simulink model "gm_uz_pmsm_model_6LUT_pd"  (R2023b)
settings: Solver=FixedStepAuto  StartTime=0.0  StopTime=0.05  RelTol=1e-3
PreLoadFcn:
  | uz_pmsm_model_init_parameter
PostLoadFcn:
  | % Import the data from Excel for a lookup table
  | FluxMapData = readtable('C:\Users\Philipp\ultrazohm\ultrazohm_sw\ip_cores\uz_pmsm_model\FluxMapData_2023-05-26_13-07-57.csv');
  | % Row indices for lookup table
  | d_current_in_d_axis = FluxMapData(8:27,1:end);
  | % Column indices for lookup table
  | q_current_in_d_axis = FluxMapData(29:48,1:end);
  | % Output values for lookup table
  | d_Flux_d_axis = FluxMapData(50:69,1:end);
undefined symbols (not defined in the file or in its folder): ad1, ad2, ad3, ad4, ad5, ad6, aq1, aq2, aq3, aq4, aq5, aq6, d_current_d_Flux, d_current_q_Flux, entkopplung_dynamic, entkopplung_linear, entkopplung_static, Fid1_Giq1, Fid2_Giq2, Flux_d, Flux_q, friction_coefficient, inertia, Ki_Bo_d, Ki_Bo_q, Kp_Bo_d, Kp_Bo_q, L_d, L_q, Ldq, parameter_nachfuerung, polepair, praediktion_entkopplung_nonlinear, psi_pm, q_current_d_Flux, q_current_q_Flux, R_1, simulate_mechanical, simulate_nonlinear_modell, simulate_open_loop, static_friction_torque, tau_sum, ts_regler
libraries: hdlmdlgenlib x21, slpidlib x2
(part 2 of 3)

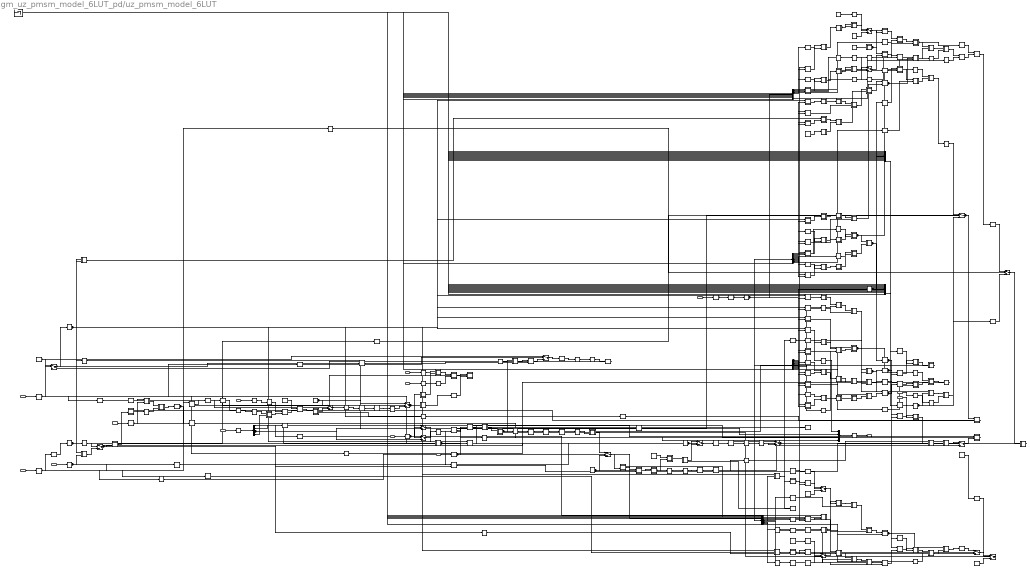
== system gm_uz_pmsm_model_6LUT_pd/uz_pmsm_model_6LUT ==
  reset_integrators : Inport  OutDataTypeStr=boolean  PortDimensions=1  SampleTime=2e-06
  simulate_mechanical : Inport  Port=2  OutDataTypeStr=boolean  PortDimensions=1  SampleTime=2e-06
  simulate_nonlinear : Inport  Port=3  OutDataTypeStr=boolean  PortDimensions=1  SampleTime=2e-06
  reciprocal_J : Inport  Port=4  OutDataTypeStr=single  PortDimensions=1  SampleTime=2e-06
  mu : Inport  Port=5  OutDataTypeStr=single  PortDimensions=1  SampleTime=2e-06
  M_n0 : Inport  Port=6  OutDataTypeStr=single  PortDimensions=1  SampleTime=2e-06
  R1 : Inport  Port=7  OutDataTypeStr=single  PortDimensions=1  SampleTime=2e-06
  polepairs : Inport  Port=8  OutDataTypeStr=single  PortDimensions=1  SampleTime=2e-06
  Ld : Inport  Port=9  OutDataTypeStr=single  PortDimensions=1  SampleTime=2e-06
  Lq : Inport  Port=10  OutDataTypeStr=single  PortDimensions=1  SampleTime=2e-06
  psi_pm : Inport  Port=11  OutDataTypeStr=single  PortDimensions=1  SampleTime=2e-06
  fitting_parameters : Inport  Port=12  OutDataTypeStr=single  PortDimensions=[14]  SampleTime=2e-06
  inputs : Inport  Port=13  OutDataTypeStr=single  PortDimensions=[4]  SampleTime=2e-06
  Abs : Subsystem
      mask Display: disp('NFP\nabs');
  Constant : Constant  Value=double(0.5)  OutDataTypeStr=double  SampleTime=1e-08
  Constant1 : Constant  Value=double(1)  OutDataTypeStr=double  SampleTime=1e-08
  Constant11 : Constant  Value=double(1)  OutDataTypeStr=double  SampleTime=1e-08
  Data Type Conversion{11,15..17} (4 alike) : DataTypeConversion  OutDataTypeStr=single
  Data Type Conversion171 : Subsystem
      mask Display: disp('NFP\nconv');
  Data Type Conversion172 : Subsystem
      mask Display: disp('NFP\nconv');
  Data Type Conversion173 : Subsystem
      mask Display: disp('NFP\nconv');
  Data Type Conversion17_to_const : Constant  Value=double(0)  OutDataTypeStr=single  SampleTime=1e-08
  Delay : RateTransition  OutPortSampleTimeOpt=Multiple of input port sample time  OutPortSampleTimeMultiple=200
  Delay1_lowered : RateTransition  OutPortSampleTimeOpt=Multiple of input port sample time  OutPortSampleTimeMultiple=200
  Delay1_lowered1 : RateTransition  OutPortSampleTimeOpt=Multiple of input port sample time  OutPortSampleTimeMultiple=200
  Delay1_lowered2 : RateTransition  OutPortSampleTimeOpt=Multiple of input port sample time  OutPortSampleTimeMultiple=200
  Delay1_lowered_absorbed : Delay  DelayLength=0
  Delay1_lowered_absorbed1 : Delay  DelayLength=0
  Delay1_lowered_absorbed2 : Delay  DelayLength=0
  Delay_absorbed : Delay  DelayLength=0
  Divide : Subsystem
      mask Display: disp('NFP\nmul');
  Divide1 : Subsystem
      mask Display: disp('NFP\nmul');
  Divide_recip : Subsystem
      mask Display: disp('NFP\nmath');
  Factor : Subsystem
      mask Display: disp('NFP\nmul');
  Factor_const : Constant  Value=single(1.5)  OutDataTypeStr=single  SampleTime=1e-08
  From1 : hdlmdlgenlib/Buffer
  From1_out1_0_term0 : Terminator
  From1_out1_10_term10 : Terminator
  From1_out1_11_term11 : Terminator
  From1_out1_12_term12 : Terminator
  From1_out1_13_term13 : Terminator
  From1_out1_1_term1 : Terminator
  From1_out1_2_term2 : Terminator
  From1_out1_3_term3 : Terminator
  From1_out1_4_term4 : Terminator
  From1_out1_5_term5 : Terminator
  From1_out1_6_term6 : Terminator
  From1_out1_7_term7 : Terminator
  From1_out1_8_term8 : Terminator
  From1_out1_9_term9 : Terminator
  From2 : hdlmdlgenlib/Buffer
  From2_out1_0_term0 : Terminator
  From2_out1_0_term01 : Terminator
  From2_out1_10_term10 : Terminator
  From2_out1_10_term101 : Terminator
  From2_out1_11_term11 : Terminator
  From2_out1_11_term111 : Terminator
  From2_out1_12_term12 : Terminator
  From2_out1_13_term13 : Terminator
  From2_out1_1_term1 : Terminator
  From2_out1_1_term11 : Terminator
  From2_out1_2_term2 : Terminator
  From2_out1_2_term21 : Terminator
  From2_out1_3_term3 : Terminator
  From2_out1_3_term31 : Terminator
  From2_out1_4_term4 : Terminator
  From2_out1_4_term41 : Terminator
  From2_out1_5_term5 : Terminator
  From2_out1_5_term51 : Terminator
  From2_out1_6_term6 : Terminator
  From2_out1_6_term61 : Terminator
  From2_out1_7_term7 : Terminator
  From2_out1_7_term71 : Terminator
  From2_out1_8_term8 : Terminator
  From2_out1_8_term81 : Terminator
  From2_out1_9_term9 : Terminator
  From2_out1_9_term91 : Terminator
  From3 : hdlmdlgenlib/Buffer
  Gain : Subsystem
      mask Display: disp('NFP\nmul');
  Gain7 : Subsystem
      mask Display: disp('NFP\nmul');
  Gain71 : Subsystem
      mask Display: disp('NFP\nmul');
  Gain7_const : Constant  Value=single(2e-06)  OutDataTypeStr=single  SampleTime=1e-08
  Gain7_const1 : Constant  Value=single(2e-06)  OutDataTypeStr=single  SampleTime=1e-08
  Gain_const : Constant  Value=single(2e-06)  OutDataTypeStr=single  SampleTime=1e-08
  Gain_unaryminus : Subsystem
      mask Display: disp('NFP\numinus');
  Gain_unaryminus1 : Subsystem
      mask Display: disp('NFP\numinus');
  Goto1 : hdlmdlgenlib/Buffer
  Goto2 : hdlmdlgenlib/Buffer
  Initial_Val : Constant  Value=single(0)  OutDataTypeStr=single  SampleTime=1e-08
  Initial_Val1 : Constant  Value=single(0)  OutDataTypeStr=single  SampleTime=1e-08
  Initial_Val2 : Constant  Value=single(0)  OutDataTypeStr=single  SampleTime=1e-08
  Ldd : hdlmdlgenlib/Buffer
  Log : Subsystem
      mask Display: disp('NFP\nmath');
  Log1 : Subsystem
      mask Display: disp('NFP\nmath');
  Log11 : Subsystem
      mask Display: disp('NFP\nmath');
  Log2 : Subsystem
      mask Display: disp('NFP\nmath');
  Lqq : hdlmdlgenlib/Buffer
  M_Mi : hdlmdlgenlib/Buffer
  Product : Subsystem
      mask Display: disp('NFP\nmul');
  Product1 : Subsystem
      mask Display: disp('NFP\nmul');
  Product10 : Subsystem
      mask Display: disp('NFP\nmul');
  Product101 : Subsystem
      mask Display: disp('NFP\nmul');
  Product102 : Subsystem
      mask Display: disp('NFP\nmul');
  Product103 : Subsystem
      mask Display: disp('NFP\nmul');
  Product104 : Subsystem
      mask Display: disp('NFP\nmul');
  Product11 : Subsystem
      mask Display: disp('NFP\nmul');
  Product110 : Subsystem
      mask Display: disp('NFP\nmul');
  Product111 : Subsystem
      mask Display: disp('NFP\nmul');
  Product112 : Subsystem
      mask Display: disp('NFP\nmul');
  Product113 : Subsystem
      mask Display: disp('NFP\nmul');
  Product12 : Subsystem
      mask Display: disp('NFP\nmul');
  Product121 : Subsystem
      mask Display: disp('NFP\nmul');
  Product122 : Subsystem
      mask Display: disp('NFP\nmul');
  Product13 : Subsystem
      mask Display: disp('NFP\nmul');
  Product131 : Subsystem
      mask Display: disp('NFP\nmul');
  Product132 : Subsystem
      mask Display: disp('NFP\nmul');
  Product133 : Subsystem
      mask Display: disp('NFP\nmul');
  Product14 : Subsystem
      mask Display: disp('NFP\nmul');
  Product141 : Subsystem
      mask Display: disp('NFP\nmul');
  Product15 : Subsystem
      mask Display: disp('NFP\nmul');
  Product151 : Subsystem
      mask Display: disp('NFP\nmul');
  Product16 : Subsystem
      mask Display: disp('NFP\nmul');
  Product161 : Subsystem
      mask Display: disp('NFP\nmul');
  Product162 : Subsystem
      mask Display: disp('NFP\nmul');
  Product17 : Subsystem
      mask Display: disp('NFP\nmul');
  Product18 : Subsystem
      mask Display: disp('NFP\nmul');
  Product19 : Subsystem
      mask Display: disp('NFP\nmul');
  Product2 : Subsystem
      mask Display: disp('NFP\nmul');
  Product20 : Subsystem
      mask Display: disp('NFP\nmul');
  Product201 : Subsystem
      mask Display: disp('NFP\nmul');
  Product202 : Subsystem
      mask Display: disp('NFP\nmul');
  Product203 : Subsystem
      mask Display: disp('NFP\nmul');
  Product204 : Subsystem
      mask Display: disp('NFP\nmul');
  Product205 : Subsystem
      mask Display: disp('NFP\nmul');
  Product206 : Subsystem
      mask Display: disp('NFP\nmul');
  Product207 : Subsystem
      mask Display: disp('NFP\nmul');
  Product21 : Subsystem
      mask Display: disp('NFP\nmul');
  Product211 : Subsystem
      mask Display: disp('NFP\nmul');
  Product22 : Subsystem
      mask Display: disp('NFP\nmul');
  Product23 : Subsystem
      mask Display: disp('NFP\nmul');
  Product24 : Subsystem
      mask Display: disp('NFP\nmul');
  Product25 : Subsystem
      mask Display: disp('NFP\nmul');
  Product26 : Subsystem
      mask Display: disp('NFP\nmul');
  Product3 : Subsystem
      mask Display: disp('NFP\nmul');
  Product31 : Subsystem
      mask Display: disp('NFP\nmul');
  Product32 : Subsystem
      mask Display: disp('NFP\nmul');
  Product33 : Subsystem
      mask Display: disp('NFP\nmul');
  Product34 : Subsystem
      mask Display: disp('NFP\nmul');
  Product35 : Subsystem
      mask Display: disp('NFP\nmul');
  Product36 : Subsystem
      mask Display: disp('NFP\nmul');
  Product37 : Subsystem
      mask Display: disp('NFP\nmul');
  Product4 : Subsystem
      mask Display: disp('NFP\nmul');
  Product41 : Subsystem
      mask Display: disp('NFP\nmul');
  Product42 : Subsystem
      mask Display: disp('NFP\nmul');
  Product43 : Subsystem
      mask Display: disp('NFP\nmul');
  Product44 : Subsystem
      mask Display: disp('NFP\nmul');
  Product5 : Subsystem
      mask Display: disp('NFP\nmul');
  Product51 : Subsystem
      mask Display: disp('NFP\nmul');
  Product52 : Subsystem
      mask Display: disp('NFP\nmul');
  Product6 : Subsystem
      mask Display: disp('NFP\nmul');
  Product61 : Subsystem
      mask Display: disp('NFP\nmul');
  Product7 : Subsystem
      mask Display: disp('NFP\nmul');
  Product71 : Subsystem
      mask Display: disp('NFP\nmul');
  Product72 : Subsystem
      mask Display: disp('NFP\nmul');
  Product8 : Subsystem
      mask Display: disp('NFP\nmul');
  Product81 : Subsystem
      mask Display: disp('NFP\nmul');
  Product9 : Subsystem
      mask Display: disp('NFP\nmul');
  Product91 : Subsystem
      mask Display: disp('NFP\nmul');
  Product92 : Subsystem
      mask Display: disp('NFP\nmul');
  Product93 : Subsystem
      mask Display: disp('NFP\nmul');
  Sign1 : Subsystem
      mask Display: disp('NFP\nsignum');
  Sum : Subsystem
      mask Display: disp('NFP\nadd');
  Sum1 : Subsystem
      mask Display: disp('NFP\nadd');
  Sum10 : Subsystem
      mask Display: disp('NFP\nadd');
  Sum101 : Subsystem
      mask Display: disp('NFP\nadd');
  Sum11 : Subsystem
      mask Display: disp('NFP\nadd');
  Sum12 : Subsystem
      mask Display: disp('NFP\nadd');
  Sum13 : Subsystem
      mask Display: disp('NFP\nadd');
  Sum14 : Subsystem
      mask Display: disp('NFP\nadd');
  Sum2 : Subsystem
      mask Display: disp('NFP\nadd');
  Sum21 : Subsystem
      mask Display: disp('NFP\nadd');
  Sum22 : Subsystem
      mask Display: disp('NFP\nadd');
  Sum23 : Subsystem
      mask Display: disp('NFP\nadd');
  Sum3 : Subsystem
      mask Display: disp('NFP\nadd');
  Sum31 : Subsystem
      mask Display: disp('NFP\nadd');
  Sum32 : Subsystem
      mask Display: disp('NFP\nadd');
  Sum33 : Subsystem
      mask Display: disp('NFP\nadd');
  Sum3_stage2 : Subsystem
      mask Display: disp('NFP\nadd');
  Sum3_stage21 : Subsystem
      mask Display: disp('NFP\nadd');
  Sum3_stage3 : Subsystem
      mask Display: disp('NFP\nadd');
  Sum3_stage31 : Subsystem
      mask Display: disp('NFP\nadd');
  Sum3_stage4 : Subsystem
      mask Display: disp('NFP\nadd');
  Sum4 : Subsystem
      mask Display: disp('NFP\nadd');
  Sum41 : Subsystem
      mask Display: disp('NFP\nadd');
  Sum42 : Subsystem
      mask Display: disp('NFP\nadd');
  Sum43 : Subsystem
      mask Display: disp('NFP\nadd');
  Sum4_stage2 : Subsystem
      mask Display: disp('NFP\nadd');
  Sum4_stage3 : Subsystem
      mask Display: disp('NFP\nadd');
  Sum4_stage4 : Subsystem
      mask Display: disp('NFP\nadd');
  Sum5 : Subsystem
      mask Display: disp('NFP\nadd');
  Sum51 : Subsystem
      mask Display: disp('NFP\nadd');
  Sum52 : Subsystem
      mask Display: disp('NFP\nadd');
  Sum53 : Subsystem
      mask Display: disp('NFP\nadd');
  Sum6 : Subsystem
      mask Display: disp('NFP\nadd');
  Sum7 : Subsystem
      mask Display: disp('NFP\nadd');
  Sum71 : Subsystem
      mask Display: disp('NFP\nadd');
  Sum8 : Subsystem
      mask Display: disp('NFP\nadd');
  Switch{,1..6,11} (8 alike) : Switch  Criteria=u2 ~= 0  Threshold=double(0)  OutDataTypeStr=single  SampleTime=1e-08  SaturateOnIntegerOverflow=off  InputSameDT=off
  Tanh : Subsystem
      mask Display: disp('NFP\ntrig');
  Tanh1 : Subsystem
      mask Display: disp('NFP\ntrig');
  Tanh11 : Subsystem
      mask Display: disp('NFP\ntrig');
  Tanh12 : Subsystem
      mask Display: disp('NFP\ntrig');
  Tanh13 : Subsystem
      mask Display: disp('NFP\ntrig');
  Tanh2 : Subsystem
      mask Display: disp('NFP\ntrig');
  Tanh21 : Subsystem
      mask Display: disp('NFP\ntrig');
  Tanh3 : Subsystem
      mask Display: disp('NFP\ntrig');
  Tanh31 : Subsystem
      mask Display: disp('NFP\ntrig');
  Tanh4 : Subsystem
      mask Display: disp('NFP\ntrig');
  Tanh41 : Subsystem
      mask Display: disp('NFP\ntrig');
  Tanh5 : Subsystem
      mask Display: disp('NFP\ntrig');
  Unit Delay : RateTransition  OutPortSampleTimeOpt=Multiple of input port sample time  OutPortSampleTimeMultiple=200
  Unit Delay1 : RateTransition  OutPortSampleTimeOpt=Multiple of input port sample time  OutPortSampleTimeMultiple=200
  Unit Delay1_absorbed : Delay  DelayLength=0
  Unit Delay_absorbed : Delay  DelayLength=0
  crp_out_delay{,1..5} (6 alike) : Delay  DelayLength=double(1)  InitialCondition=0  SampleTime=1e-08
  default_value{,1..4} (5 alike) : Constant  Value=double(1)  OutDataTypeStr=single  SampleTime=1e-08
  delayMatch{,1..24,26..28,30..41,43..45,47..52,54..58} (54 alike) : Delay  DelayLength=double(1)  InitialCondition=0  SampleTime=1e-08
  delayMatch25 : Delay  DelayLength=double(35)  InitialCondition=0  SampleTime=1e-08
  delayMatch29 : Delay  DelayLength=double(35)  InitialCondition=0  SampleTime=1e-08
  delayMatch42 : Delay  DelayLength=double(29)  InitialCondition=0  SampleTime=1e-08
  delayMatch46 : Delay  DelayLength=double(29)  InitialCondition=0  SampleTime=1e-08
  delayMatch53 : Delay  DelayLength=double(97)  InitialCondition=0  SampleTime=1e-08
  fitting_parameters_12_term12 : Terminator
  fitting_parameters_13_term13 : Terminator
  in0_repeat : RateTransition  Integrity=off  Deterministic=off  OutPortSampleTimeOpt=Multiple of input port sample time  OutPortSampleTimeMultiple=1/200
  in10_repeat : RateTransition  Integrity=off  Deterministic=off  OutPortSampleTimeOpt=Multiple of input port sample time  OutPortSampleTimeMultiple=1/200
  in11_repeat : RateTransition  Integrity=off  Deterministic=off  OutPortSampleTimeOpt=Multiple of input port sample time  OutPortSampleTimeMultiple=1/200
  in12_repeat : RateTransition  Integrity=off  Deterministic=off  OutPortSampleTimeOpt=Multiple of input port sample time  OutPortSampleTimeMultiple=1/200
  in13_repeat : RateTransition  Integrity=off  Deterministic=off  OutPortSampleTimeOpt=Multiple of input port sample time  OutPortSampleTimeMultiple=1/200
  in14_repeat : RateTransition  Integrity=off  Deterministic=off  OutPortSampleTimeOpt=Multiple of input port sample time  OutPortSampleTimeMultiple=1/200
  in15_repeat : RateTransition  Integrity=off  Deterministic=off  OutPortSampleTimeOpt=Multiple of input port sample time  OutPortSampleTimeMultiple=1/200
  in16_repeat : RateTransition  Integrity=off  Deterministic=off  OutPortSampleTimeOpt=Multiple of input port sample time  OutPortSampleTimeMultiple=1/200
  in17_repeat : RateTransition  Integrity=off  Deterministic=off  OutPortSampleTimeOpt=Multiple of input port sample time  OutPortSampleTimeMultiple=1/200
  in18_repeat : RateTransition  Integrity=off  Deterministic=off  OutPortSampleTimeOpt=Multiple of input port sample time  OutPortSampleTimeMultiple=1/200
  in1_repeat : RateTransition  Integrity=off  Deterministic=off  OutPortSampleTimeOpt=Multiple of input port sample time  OutPortSampleTimeMultiple=1/200
  in2_repeat : RateTransition  Integrity=off  Deterministic=off  OutPortSampleTimeOpt=Multiple of input port sample time  OutPortSampleTimeMultiple=1/200
  in3_repeat : RateTransition  Integrity=off  Deterministic=off  OutPortSampleTimeOpt=Multiple of input port sample time  OutPortSampleTimeMultiple=1/200
  in4_repeat : RateTransition  Integrity=off  Deterministic=off  OutPortSampleTimeOpt=Multiple of input port sample time  OutPortSampleTimeMultiple=1/200
  in5_repeat : RateTransition  Integrity=off  Deterministic=off  OutPortSampleTimeOpt=Multiple of input port sample time  OutPortSampleTimeMultiple=1/200
  in6_repeat : RateTransition  Integrity=off  Deterministic=off  OutPortSampleTimeOpt=Multiple of input port sample time  OutPortSampleTimeMultiple=1/200
  in7_repeat : RateTransition  Integrity=off  Deterministic=off  OutPortSampleTimeOpt=Multiple of input port sample time  OutPortSampleTimeMultiple=1/200
  in8_repeat : RateTransition  Integrity=off  Deterministic=off  OutPortSampleTimeOpt=Multiple of input port sample time  OutPortSampleTimeMultiple=1/200
  in9_repeat : RateTransition  Integrity=off  Deterministic=off  OutPortSampleTimeOpt=Multiple of input port sample time  OutPortSampleTimeMultiple=1/200
  mux : Mux
  psi_d_approx : hdlmdlgenlib/Buffer
  psi_q_approx : hdlmdlgenlib/Buffer
  reset_in : Switch  Criteria=u2 ~= 0  Threshold=double(0)  OutDataTypeStr=single  SampleTime=1e-08  SaturateOnIntegerOverflow=off  InputSameDT=off
  reset_in1 : Switch  Criteria=u2 ~= 0  Threshold=double(0)  OutDataTypeStr=single  SampleTime=1e-08  SaturateOnIntegerOverflow=off  InputSameDT=off
  reset_in2 : Switch  Criteria=u2 ~= 0  Threshold=double(0)  OutDataTypeStr=single  SampleTime=1e-08  SaturateOnIntegerOverflow=off  InputSameDT=off
  reset_out : Switch  Criteria=u2 ~= 0  Threshold=double(0)  OutDataTypeStr=single  SampleTime=1e-08  SaturateOnIntegerOverflow=off  InputSameDT=off
  reset_out1 : Switch  Criteria=u2 ~= 0  Threshold=double(0)  OutDataTypeStr=single  SampleTime=1e-08  SaturateOnIntegerOverflow=off  InputSameDT=off
  reset_out2 : Switch  Criteria=u2 ~= 0  Threshold=double(0)  OutDataTypeStr=single  SampleTime=1e-08  SaturateOnIntegerOverflow=off  InputSameDT=off
  select_signal{,1..4} (5 alike) : Constant  Value=double(1)  OutDataTypeStr=boolean  SampleTime=1e-08
  t : RateTransition  OutPortSampleTimeOpt=Multiple of input port sample time  OutPortSampleTimeMultiple=200
  t{1..6} (6 alike) : Demux  Outputs=14
  t{8..18} (11 alike) : hdlmdlgenlib/Buffer
  t7 : Demux
  zero_protection{,1..4} (5 alike) : Switch  Criteria=u2 ~= 0  Threshold=double(0)  OutDataTypeStr=single  SampleTime=1e-08  SaturateOnIntegerOverflow=off  InputSameDT=off
  outputs : Outport  SampleTime=2e-06
  wires:
  reset_integrators/1 -> in8_repeat/1
  simulate_mechanical/1 -> in10_repeat/1
  simulate_nonlinear/1 -> in1_repeat/1
  reciprocal_J/1 -> in12_repeat/1
  mu/1 -> in0_repeat/1
  M_n0/1 -> in18_repeat/1
  R1/1 -> in3_repeat/1
  polepairs/1 -> in17_repeat/1
  Ld/1 -> in4_repeat/1
  Lq/1 -> in2_repeat/1
  psi_pm/1 -> in5_repeat/1
  fitting_parameters/1 -> in7_repeat/1
  inputs/1 -> in14_repeat/1
  t/1 -> outputs/1
  in0_repeat/1 -> Product122/1(In1)
  in1_repeat/1 -> delayMatch51/1, delayMatch40/1, delayMatch34/1, delayMatch33/1, Goto2/1
  in2_repeat/1 -> delayMatch52/1, Product1/2(In2)
  in3_repeat/1 -> Product43/1(In1), Product9/2(In2)
  in4_repeat/1 -> delayMatch35/1, Product5/2(In2)
  in5_repeat/1 -> delayMatch5/1
  in7_repeat/1 -> t6/1, t3/1, Goto1/1
  in8_repeat/1 -> delayMatch58/1, delayMatch55/1, delayMatch37/1, reset_out1/2, reset_out2/2, reset_out/2
  in10_repeat/1 -> Switch/2, Switch11/2
  in12_repeat/1 -> delayMatch56/1
  in14_repeat/1 -> t7/1
  in17_repeat/1 -> delayMatch15/1, Product131/2(In2)
  in18_repeat/1 -> delayMatch19/1
  mux/1 -> t/1
  Delay1_lowered/1 -> Delay1_lowered_absorbed/1
  Delay1_lowered_absorbed/1 -> in16_repeat/1
  in16_repeat/1 -> reset_out2/3
  Unit Delay1/1 -> Unit Delay1_absorbed/1
  Unit Delay1_absorbed/1 -> in15_repeat/1
  in15_repeat/1 -> delayMatch23/1
  Delay/1 -> Delay_absorbed/1
  Delay_absorbed/1 -> in13_repeat/1
  in13_repeat/1 -> Sum14/1(In1)
  Delay1_lowered1/1 -> Delay1_lowered_absorbed1/1
  Delay1_lowered_absorbed1/1 -> in11_repeat/1
  in11_repeat/1 -> reset_out1/3
  Delay1_lowered2/1 -> Delay1_lowered_absorbed2/1
  Delay1_lowered_absorbed2/1 -> in9_repeat/1
  in9_repeat/1 -> reset_out/3
  Unit Delay/1 -> Unit Delay_absorbed/1
  Unit Delay_absorbed/1 -> in6_repeat/1
  in6_repeat/1 -> delayMatch39/1
  crp_out_delay/1 -> Delay/1
  crp_out_delay1/1 -> Unit Delay/1
  crp_out_delay2/1 -> Delay1_lowered/1
  crp_out_delay3/1 -> Unit Delay1/1
  crp_out_delay4/1 -> Delay1_lowered2/1
  crp_out_delay5/1 -> Delay1_lowered1/1
  Data Type Conversion16/1 -> mux/3
  Lqq/1 -> Switch1/1
  Constant1/1 -> Data Type Conversion171/1(In1)
  Data Type Conversion171/1(Out1) -> Product133/1(In1), Product162/1(In1)
  Switch2/1 -> Divide_recip/1(In1)
  Ldd/1 -> Switch2/1
  Constant11/1 -> Data Type Conversion172/1(In1)
  Data Type Conversion172/1(Out1) -> Product132/1(In1), Product161/1(In1)
  Product31/1(Out1) -> Sum2/2(In2)
  Sum2/1(Out1) -> Product102/1(In1)
  Product21/1(Out1) -> Sum4_stage3/2(In2)
  Goto2/1 -> From3/1
  delayMatch6/1 -> Switch5/2
  Switch5/1 -> Product21/1(In1), Product37/1(In1)
  psi_d_approx/1 -> Switch5/1
  Gain_unaryminus/1(Out1) -> Product11/2(In2)
  delayMatch22/1 -> Product207/2(In2)
  Goto1/1 -> From2/1, From1/1
  From2/1 -> t2/1, t1/1
  delayMatch38/1 -> Product201/2(In2)
  Product201/1(Out1) -> Gain_unaryminus/1(In1)
  t10/1 -> Product206/1(In1), Product20/1(In1)
  Constant/1 -> Data Type Conversion173/1(In1)
  Data Type Conversion173/1(Out1) -> Product71/2(In2)
  Sum41/1(Out1) -> Product7/2(In2)
  delayMatch1/1 -> Product13/2(In2)
  delayMatch/1 -> Product4/2(In2)
  t3/3 -> Sum4/2(In2)
  delayMatch3/1 -> Product32/2(In2)
  delayMatch2/1 -> Product22/2(In2)
  t3/6 -> Sum11/2(In2)
  t3/7 -> Product93/1(In1)
  t3/8 -> Product41/2(In2), Product93/2(In2)
  t3/9 -> Sum41/1(In1)
  t3/10 -> Product113/1(In1)
  t3/11 -> Product51/2(In2), Product113/2(In2)
  t3/12 -> Sum41/2(In2)
  delayMatch4/1 -> Product101/2(In2)
  Product32/1(Out1) -> Sum21/2(In2)
  t15/1 -> Product10/1(In1)
  t14/1 -> Sum7/1(In1)
  Sum7/1(Out1) -> psi_d_approx/1
  Product101/1(Out1) -> Sum7/2(In2)
  Sum3_stage3/1(Out1) -> t8/1, Product10/2(In2)
  t8/1 -> Product102/2(In2)
  Product103/1(Out1) -> Sum71/2(In2)
  Sum71/1(Out1) -> Ldd/1
  t18/1 -> Sum71/1(In1)
  delayMatch26/1 -> Product16/2(In2)
  delayMatch24/1 -> Product/2(In2)
  t4/3 -> Sum/2(In2)
  delayMatch30/1 -> Product3/2(In2)
  delayMatch28/1 -> Product2/2(In2)
  t4/6 -> Sum1/2(In2)
  delayMatch32/1 -> Product103/2(In2)
  From1/1 -> t5/1, t4/1
  delayMatch43/1 -> Product19/2(In2)
  delayMatch44/1 -> Product110/2(In2)
  delayMatch45/1 -> Sum12/2(In2)
  delayMatch47/1 -> Product34/2(In2)
  delayMatch48/1 -> Product35/2(In2)
  delayMatch49/1 -> Sum42/2(In2)
  delayMatch50/1 -> Product205/2(In2)
  Product110/1(Out1) -> Sum12/1(In1)
  Sum10/1(Out1) -> Lqq/1
  Sum31/1(Out1) -> Product72/2(In2)
  Product72/1(Out1) -> Tanh41/1(In1)
  Sum6/1(Out1) -> Product104/2(In2)
  Product104/1(Out1) -> Tanh21/1(In1)
  Product33/1(Out1) -> Sum13/1(In1)
  t6/1 -> Product211/1(In1)
  delayMatch9/1 -> Product72/1(In1)
  t6/3 -> Sum31/2(In2)
  t6/4 -> Product81/1(In1)
  delayMatch10/1 -> Product104/1(In1)
  t6/6 -> Sum6/2(In2)
  delayMatch7/1 -> Product111/2(In2)
  t6/8 -> Product23/2(In2)
  t6/9 -> Product52/2(In2)
  delayMatch8/1 -> Product33/2(In2)
  t6/11 -> Product24/2(In2)
  t6/12 -> Product61/2(In2)
  delayMatch11/1 -> Product203/2(In2)
  Product203/1(Out1) -> Sum101/2(In2)
  Sum5/1(Out1) -> t9/1, Product202/2(In2)
  t9/1 -> Product204/2(In2)
  Product205/1(Out1) -> Sum10/2(In2)
  Product35/1(Out1) -> Sum42/1(In1)
  t11/1 -> Product25/1(In1), Product24/1(In1), Product61/1(In1), Product52/1(In1), Product23/1(In1), Product18/1(In1), Product51/1(In1), Product8/2(In2), Product8/1(In1), Product41/1(In1), Product9/1(In1), Product1/1(In1), delayMatch13/1, Data Type Conversion15/1
  delayMatch54/1 -> Sum51/2(In2)
  Initial_Val/1 -> reset_out/1, reset_in/1
  reset_in/1 -> crp_out_delay4/1
  Gain7/1(Out1) -> Sum51/1(In1)
  Divide1/1(Out1) -> Gain7/2(In2), crp_out_delay3/1
  delayMatch18/1 -> mux/4
  Switch11/1 -> Data Type Conversion17/1
  delayMatch57/1 -> Sum32/2(In2)
  Initial_Val1/1 -> reset_out1/1, reset_in1/1
  reset_in1/1 -> crp_out_delay5/1
  delayMatch21/1 -> Sum3_stage21/1(In1)
  delayMatch41/1 -> Sum4_stage2/1(In1)
  t7/3 -> Switch/3, Switch11/3
  t7/4 -> Sum14/2(In2)
  Switch4/1 -> Sum4_stage2/2(In2)
  Data Type Conversion17_to_const/1 -> Switch3/3, Switch4/3
  Switch3/1 -> Sum3_stage31/2(In2)
  Gain_unaryminus1/1(Out1) -> Product121/1(In1)
  Product207/1(Out1) -> Gain_unaryminus1/1(In1)
  t12/1 -> Product206/2(In2), Product20/2(In2)
  t16/1 -> Product202/1(In1)
  t17/1 -> Sum101/1(In1)
  Sum101/1(Out1) -> psi_q_approx/1
  psi_q_approx/1 -> Switch6/1
  Switch6/1 -> Product36/2(In2), Product26/2(In2)
  delayMatch14/1 -> Product26/1(In1)
  t13/1 -> Product43/2(In2), Sum6/1(In1), Sum31/1(In1), Sum11/1(In1), Sum4/1(In1), Product5/1(In1), Sum1/1(In1), Sum/1(In1), delayMatch14/1, Data Type Conversion11/1
  delayMatch36/1 -> Sum52/2(In2)
  Initial_Val2/1 -> reset_out2/1, reset_in2/1
  reset_in2/1 -> crp_out_delay2/1
  Gain71/1(Out1) -> Sum52/1(In1)
  Divide/1(Out1) -> Gain71/2(In2), crp_out_delay1/1
  Product36/1(Out1) -> Sum3_stage4/2(In2)
  Switch/1 -> Product131/1(In1)
  delayMatch20/1 -> Product44/2(In2)
  M_Mi/1 -> Sum8/1(In1), Data Type Conversion16/1
  Product92/1(Out1) -> M_Mi/1
  Factor/1(Out1) -> Product92/1(In1)
  delayMatch13/1 -> Product37/2(In2)
  delayMatch17/1 -> mux/2
  delayMatch16/1 -> mux/1
  delayMatch33/1 -> Switch3/2
  delayMatch52/1 -> Switch1/3
  delayMatch35/1 -> Switch2/3
  delayMatch5/1 -> Sum3/2(In2)
  delayMatch39/1 -> Product11/1(In1)
  delayMatch37/1 -> reset_in2/2
  delayMatch56/1 -> Product112/1(In1)
  delayMatch23/1 -> Product121/2(In2)
  delayMatch15/1 -> Product92/2(In2)
  delayMatch19/1 -> Sum53/2(In2)
  t1/1 -> From2_out1_0_term0/1
  t1/2 -> From2_out1_1_term1/1
  t1/3 -> From2_out1_2_term2/1
  t1/4 -> From2_out1_3_term3/1
  t1/5 -> From2_out1_4_term4/1
  t1/6 -> From2_out1_5_term51/1
  t1/7 -> From2_out1_6_term6/1
  t1/8 -> From2_out1_7_term7/1
  t1/9 -> From2_out1_8_term8/1
  t1/10 -> From2_out1_9_term9/1
  t1/11 -> From2_out1_10_term10/1
  t1/12 -> From2_out1_11_term111/1
  t1/13 -> delayMatch22/1
  t1/14 -> From2_out1_13_term13/1
  t2/1 -> From2_out1_0_term01/1
  t2/2 -> From2_out1_1_term11/1
  t2/3 -> From2_out1_2_term21/1
  t2/4 -> From2_out1_3_term31/1
  t2/5 -> From2_out1_4_term41/1
  t2/6 -> From2_out1_5_term5/1
  t2/7 -> From2_out1_6_term61/1
  t2/8 -> From2_out1_7_term71/1
  t2/9 -> From2_out1_8_term81/1
  t2/10 -> From2_out1_9_term91/1
  t2/11 -> From2_out1_10_term101/1
  t2/12 -> From2_out1_11_term11/1
  t2/13 -> From2_out1_12_term12/1
  t2/14 -> delayMatch38/1
  t3/1 -> delayMatch1/1
  t3/2 -> delayMatch/1
  t3/4 -> delayMatch3/1
  t3/5 -> delayMatch2/1
  t3/13 -> delayMatch4/1
  t3/14 -> fitting_parameters_13_term13/1
  t4/1 -> delayMatch26/1
  t4/2 -> delayMatch27/1, delayMatch24/1
  t4/4 -> delayMatch30/1
  t4/5 -> delayMatch31/1, delayMatch28/1
  t4/7 -> From1_out1_6_term6/1
  t4/8 -> From1_out1_7_term7/1
  t4/9 -> From1_out1_8_term8/1
  t4/10 -> From1_out1_9_term9/1
  t4/11 -> From1_out1_10_term10/1
  t4/12 -> From1_out1_11_term11/1
  t4/13 -> delayMatch32/1
  t4/14 -> From1_out1_13_term13/1
  t5/1 -> From1_out1_0_term0/1
  t5/2 -> From1_out1_1_term1/1
  t5/3 -> From1_out1_2_term2/1
  t5/4 -> From1_out1_3_term3/1
  t5/5 -> From1_out1_4_term4/1
  t5/6 -> From1_out1_5_term5/1
  t5/7 -> delayMatch43/1
  t5/8 -> delayMatch44/1, Product18/2(In2)
  t5/9 -> delayMatch45/1
  t5/10 -> delayMatch47/1
  t5/11 -> delayMatch48/1, Product25/2(In2)
  t5/12 -> delayMatch49/1
  t5/13 -> From1_out1_12_term12/1
  t5/14 -> delayMatch50/1
  t6/2 -> delayMatch9/1, Product211/2(In2)
  t6/5 -> delayMatch10/1, Product81/2(In2)
  t6/7 -> delayMatch7/1
  t6/10 -> delayMatch8/1
  t6/13 -> fitting_parameters_12_term12/1
  t6/14 -> delayMatch11/1
  t7/1 -> delayMatch21/1
  t7/2 -> delayMatch41/1
  Gain7_const/1 -> Gain7/1(In1)
  Gain_const/1 -> Gain/1(In1)
  Gain7_const1/1 -> Gain71/1(In1)
  Factor_const/1 -> Factor/1(In1)
  Product1/1(Out1) -> Switch6/3
  Product9/1(Out1) -> Sum4_stage4/2(In2)
  Sum/1(Out1) -> Product/1(In1)
  Product/1(Out1) -> Tanh4/1(In1)
  Tanh4/1(Out1) -> Product14/2(In2), Product14/1(In1)
  Product14/1(Out1) -> zero_protection/1
  Product132/1(Out1) -> Product16/1(In1)
  Sum1/1(Out1) -> Product2/1(In1)
  Product2/1(Out1) -> Tanh1/1(In1)
  Tanh1/1(Out1) -> Product15/2(In2), Product15/1(In1)
  Product15/1(Out1) -> zero_protection1/1
  Product161/1(Out1) -> Product3/1(In1)
  Product3/1(Out1) -> Product31/1(In1)
  Product5/1(Out1) -> Sum3/1(In1)
  Sum3/1(Out1) -> Switch5/3
  Product11/1(Out1) -> Switch4/1
  Product20/1(Out1) -> Product201/1(In1)
  Tanh/1(Out1) -> Product13/1(In1)
  Sum4/1(Out1) -> Product4/1(In1)
  Product4/1(Out1) -> Tanh/1(In1)
  Product41/1(Out1) -> Tanh2/1(In1)
  Tanh2/1(Out1) -> Log/1(In1)
  Log/1(Out1) -> Product6/1(In1)
  Product6/1(Out1) -> Sum3_stage2/1(In1)
  Product93/1(Out1) -> Product6/2(In2)
  Product8/1(Out1) -> Product7/1(In1)
  Product7/1(Out1) -> Product71/1(In1)
  Product71/1(Out1) -> Sum3_stage2/2(In2)
  Product51/1(Out1) -> Tanh3/1(In1)
  Tanh3/1(Out1) -> Log1/1(In1)
  Log1/1(Out1) -> Product12/1(In1)
  Product12/1(Out1) -> Sum3_stage3/2(In2)
  Product113/1(Out1) -> Product12/2(In2)
  Sum11/1(Out1) -> Product22/1(In1)
  Product22/1(Out1) -> Tanh11/1(In1)
  Tanh11/1(Out1) -> Product32/1(In1)
  Sum21/1(Out1) -> t15/1, t10/1
  Product13/1(Out1) -> t14/1, Sum21/1(In1)
  Product10/1(Out1) -> Product101/1(In1)
  Sum3_stage2/1(Out1) -> Sum3_stage3/1(In1)
  Product102/1(Out1) -> Product103/1(In1)
  Product16/1(Out1) -> Product17/1(In1)
  Product17/1(Out1) -> t18/1, Sum2/1(In1)
  Product18/1(Out1) -> Tanh31/1(In1)
  Tanh31/1(Out1) -> Product141/2(In2), Product141/1(In1)
  Product141/1(Out1) -> zero_protection2/1
  Product133/1(Out1) -> Product19/1(In1)
  Product19/1(Out1) -> Product110/1(In1)
  Sum12/1(Out1) -> Sum22/1(In1), Sum10/1(In1)
  Tanh41/1(Out1) -> Log2/1(In1)
  Log2/1(Out1) -> Product42/2(In2)
  Product42/1(Out1) -> Sum5/1(In1)
  Product211/1(Out1) -> Product42/1(In1)
  Tanh21/1(Out1) -> Log11/1(In1)
  Log11/1(Out1) -> Product91/2(In2)
  Product91/1(Out1) -> Sum5/2(In2)
  Product81/1(Out1) -> Product91/1(In1)
  Product23/1(Out1) -> Tanh5/1(In1)
  Tanh5/1(Out1) -> Product111/1(In1)
  Product111/1(Out1) -> Sum43/2(In2)
  Product52/1(Out1) -> Sum43/1(In1)
  Product61/1(Out1) -> Sum13/2(In2)
  Sum13/1(Out1) -> Sum23/2(In2)
  Product24/1(Out1) -> Tanh12/1(In1)
  Tanh12/1(Out1) -> Product33/1(In1)
  Product202/1(Out1) -> Product203/1(In1)
  Product204/1(Out1) -> Product205/1(In1)
  Sum22/1(Out1) -> Product204/1(In1)
  Sum42/1(Out1) -> Sum22/2(In2)
  Product34/1(Out1) -> Product35/1(In1)
  Product162/1(Out1) -> Product34/1(In1)
  Product151/1(Out1) -> zero_protection3/1
  Tanh13/1(Out1) -> Product151/2(In2), Product151/1(In1)
  Product25/1(Out1) -> Tanh13/1(In1)
  Sum51/1(Out1) -> reset_in/3
  Sum32/1(Out1) -> reset_in1/3
  Product112/1(Out1) -> Gain/2(In2)
  Sum14/1(Out1) -> Product112/2(In2)
  Sum4_stage2/1(Out1) -> Sum4_stage3/1(In1)
  Sum4_stage3/1(Out1) -> Sum4_stage4/1(In1)
  Sum4_stage4/1(Out1) -> Divide1/1(In1)
  Product121/1(Out1) -> Switch3/1
  Product206/1(Out1) -> Product207/1(In1)
  Sum23/1(Out1) -> t16/1, t12/1
  Sum43/1(Out1) -> t17/1, Sum23/1(In1)
  Product26/1(Out1) -> Sum33/2(In2)
  Product43/1(Out1) -> Sum3_stage21/2(In2)
  Sum52/1(Out1) -> reset_in2/3
  Divide_recip/1(Out1) -> Divide/2(In2)
  Sum3_stage21/1(Out1) -> Sum3_stage31/1(In1)
  Sum3_stage31/1(Out1) -> Sum3_stage4/1(In1)
  Sum3_stage4/1(Out1) -> Divide/1(In1)
  Product131/1(Out1) -> Product36/1(In1), Product21/2(In2)
  Sign1/1(Out1) -> delayMatch20/1
  Abs/1(Out1) -> Product122/2(In2)
  Product122/1(Out1) -> Sum53/1(In1)
  Sum53/1(Out1) -> Product44/1(In1)
  Product44/1(Out1) -> Sum8/2(In2)
  Sum8/1(Out1) -> crp_out_delay/1
  Sum33/1(Out1) -> Factor/2(In2)
  Product37/1(Out1) -> Sum33/1(In1)
  Gain/1(Out1) -> Sum32/1(In1)
  delayMatch25/1 -> zero_protection/2
  delayMatch29/1 -> zero_protection1/2
  delayMatch42/1 -> zero_protection2/2
  delayMatch46/1 -> zero_protection3/2
  delayMatch53/1 -> zero_protection4/2
  delayMatch12/1 -> Switch6/2
  From3/1 -> delayMatch12/1, delayMatch6/1
  Data Type Conversion11/1 -> delayMatch16/1
  Data Type Conversion15/1 -> delayMatch17/1
  Data Type Conversion17/1 -> delayMatch18/1
  delayMatch27/1 -> Product17/2(In2)
  select_signal/1 -> delayMatch25/1
  delayMatch31/1 -> Product31/2(In2)
  select_signal1/1 -> delayMatch29/1
  delayMatch34/1 -> Switch2/2
  delayMatch40/1 -> Switch4/2
  reset_out2/1 -> t13/1, delayMatch36/1
  delayMatch55/1 -> reset_in/2
  delayMatch51/1 -> Switch1/2
  select_signal2/1 -> delayMatch42/1
  select_signal3/1 -> delayMatch46/1
  Switch1/1 -> zero_protection4/1
  select_signal4/1 -> delayMatch53/1
  reset_out/1 -> t11/1, delayMatch54/1
  delayMatch58/1 -> reset_in1/2
  reset_out1/1 -> delayMatch57/1, Abs/1(In1), Sign1/1(In1), Switch/1, Switch11/1
  zero_protection/1 -> Product132/2(In2)
  default_value/1 -> zero_protection/3
  zero_protection1/1 -> Product161/2(In2)
  default_value1/1 -> zero_protection1/3
  zero_protection2/1 -> Product133/2(In2)
  default_value2/1 -> zero_protection2/3
  zero_protection3/1 -> Product162/2(In2)
  default_value3/1 -> zero_protection3/3
  zero_protection4/1 -> Divide1/2(In2)
  default_value4/1 -> zero_protection4/3

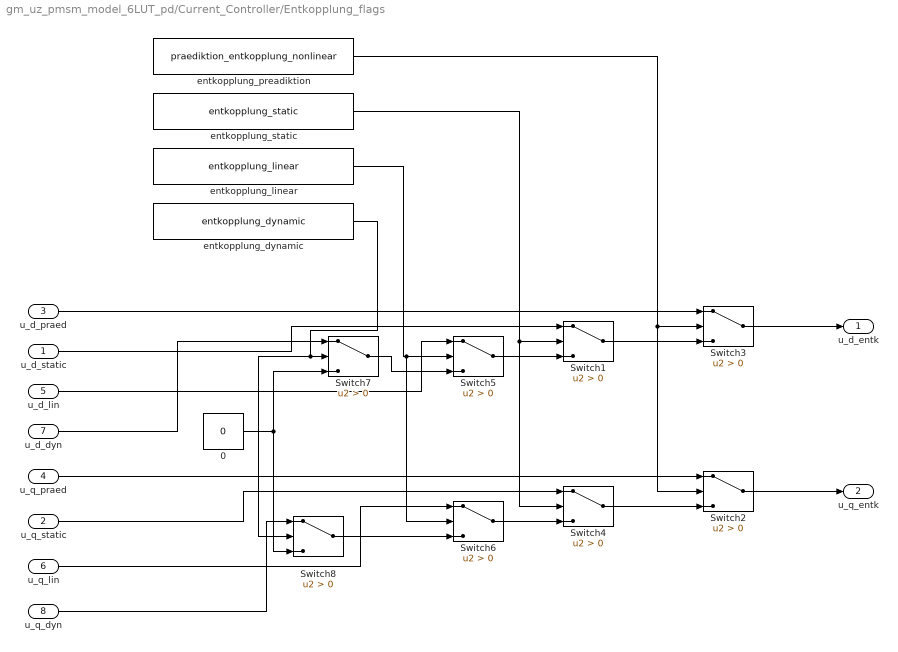
== system gm_uz_pmsm_model_6LUT_pd/Current_Controller/Entkopplung_flags ==
  u_d_static : Inport
  u_q_static : Inport  Port=2
  u_d_praed : Inport  Port=3
  u_q_praed : Inport  Port=4
  u_d_lin : Inport  Port=5
  u_q_lin : Inport  Port=6
  u_d_dyn : Inport  Port=7
  u_q_dyn : Inport  Port=8
  0 : Constant  Value=0
  Switch{1..8} (8 alike) : Switch  Criteria=u2 > Threshold  SaturateOnIntegerOverflow=off  InputSameDT=off
  entkopplung_dynamic : Constant  Value=entkopplung_dynamic
  entkopplung_linear : Constant  Value=entkopplung_linear
  entkopplung_preadiktion : Constant  Value=praediktion_entkopplung_nonlinear
  entkopplung_static : Constant  Value=entkopplung_static
  u_d_entk : Outport
  u_q_entk : Outport  Port=2
  wires:
  Switch7/1 -> Switch5/3
  u_q_dyn/1 -> Switch8/1
  Switch8/1 -> Switch6/3
  u_d_dyn/1 -> Switch7/1
  u_q_lin/1 -> Switch6/1
  u_q_static/1 -> Switch4/1
  Switch6/1 -> Switch4/3
  0/1 -> Switch7/3, Switch8/3
  entkopplung_dynamic/1 -> Switch7/2, Switch8/2
  entkopplung_linear/1 -> Switch5/2, Switch6/2
  Switch5/1 -> Switch1/3
  u_d_lin/1 -> Switch5/1
  u_d_static/1 -> Switch1/1
  entkopplung_static/1 -> Switch1/2, Switch4/2
  u_q_praed/1 -> Switch2/1
  Switch2/1 -> u_q_entk/1
  u_d_praed/1 -> Switch3/1
  Switch1/1 -> Switch3/3
  entkopplung_preadiktion/1 -> Switch3/2, Switch2/2
  Switch4/1 -> Switch2/3
  Switch3/1 -> u_d_entk/1

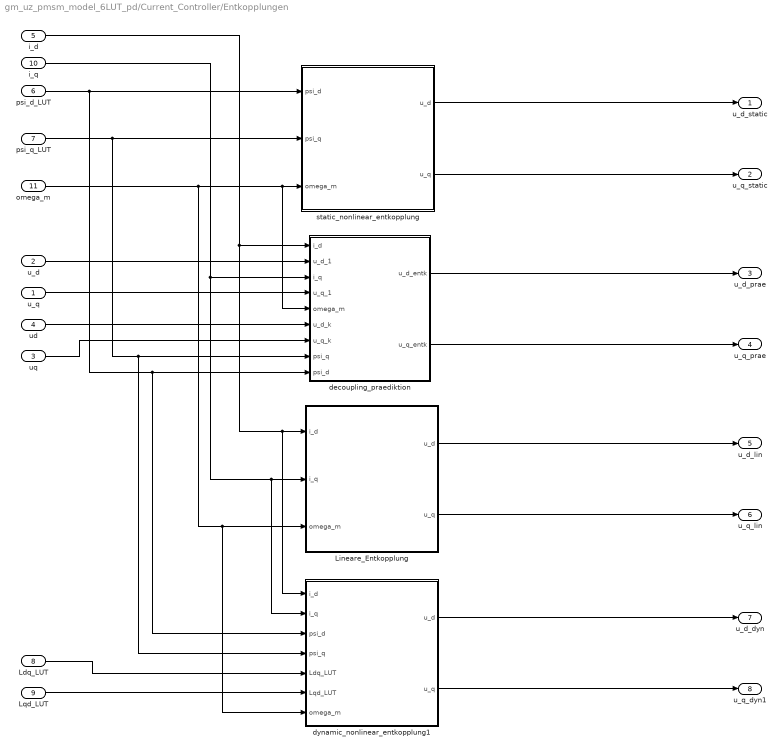
== system gm_uz_pmsm_model_6LUT_pd/Current_Controller/Entkopplungen ==
  u_q : Inport
  u_d : Inport  Port=2
  uq : Inport  Port=3
  ud : Inport  Port=4
  i_d : Inport  Port=5
  psi_d_LUT : Inport  Port=6
  psi_q_LUT : Inport  Port=7
  Ldq_LUT : Inport  Port=8
  Lqd_LUT : Inport  Port=9
  i_q : Inport  Port=10
  omega_m : Inport  Port=11
  Lineare_Entkopplung : Subsystem
  decoupling_praediktion : Subsystem
  dynamic_nonlinear_entkopplung1 : Subsystem
  static_nonlinear_entkopplung : Subsystem
  u_d_static : Outport
  u_q_static : Outport  Port=2
  u_d_prae : Outport  Port=3
  u_q_prae : Outport  Port=4
  u_d_lin : Outport  Port=5
  u_q_lin : Outport  Port=6
  u_d_dyn : Outport  Port=7
  u_q_dyn1 : Outport  Port=8
  wires:
  Lqd_LUT/1 -> dynamic_nonlinear_entkopplung1/6(Lqd_LUT)
  Ldq_LUT/1 -> dynamic_nonlinear_entkopplung1/5(Ldq_LUT)
  dynamic_nonlinear_entkopplung1/2(u_q) -> u_q_dyn1/1
  dynamic_nonlinear_entkopplung1/1(u_d) -> u_d_dyn/1
  decoupling_praediktion/2(u_q_entk) -> u_q_prae/1
  Lineare_Entkopplung/2(u_q) -> u_q_lin/1
  decoupling_praediktion/1(u_d_entk) -> u_d_prae/1
  static_nonlinear_entkopplung/2(u_q) -> u_q_static/1
  Lineare_Entkopplung/1(u_d) -> u_d_lin/1
  static_nonlinear_entkopplung/1(u_d) -> u_d_static/1
  u_d/1 -> decoupling_praediktion/2(u_d_1)
  uq/1 -> decoupling_praediktion/7(u_q_k)
  ud/1 -> decoupling_praediktion/6(u_d_k)
  i_q/1 -> decoupling_praediktion/3(i_q), Lineare_Entkopplung/2(i_q), dynamic_nonlinear_entkopplung1/2(i_q)
  i_d/1 -> decoupling_praediktion/1(i_d), Lineare_Entkopplung/1(i_d), dynamic_nonlinear_entkopplung1/1(i_d)
  u_q/1 -> decoupling_praediktion/4(u_q_1)
  psi_q_LUT/1 -> static_nonlinear_entkopplung/2(psi_q), decoupling_praediktion/8(psi_q), dynamic_nonlinear_entkopplung1/4(psi_q)
  omega_m/1 -> decoupling_praediktion/5(omega_m), static_nonlinear_entkopplung/3(omega_m), Lineare_Entkopplung/3(omega_m), dynamic_nonlinear_entkopplung1/7(omega_m)
  psi_d_LUT/1 -> decoupling_praediktion/9(psi_d), dynamic_nonlinear_entkopplung1/3(psi_d), static_nonlinear_entkopplung/1(psi_d)

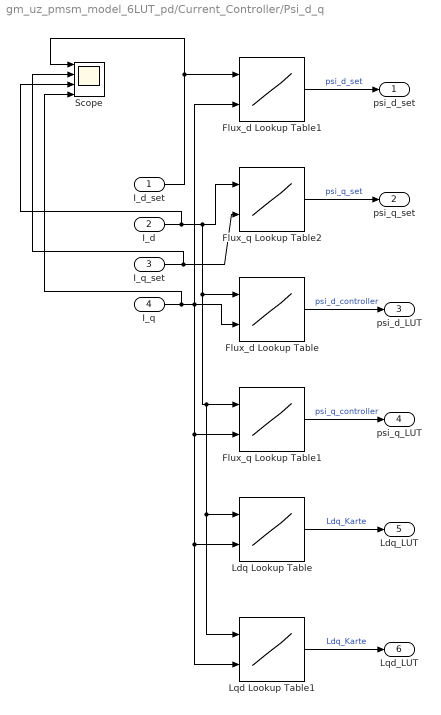
== system gm_uz_pmsm_model_6LUT_pd/Current_Controller/Psi_d_q ==
  I_d_set : Inport
  I_d : Inport  Port=2
  I_q_set : Inport  Port=3
  I_q : Inport  Port=4
  Flux_d Lookup Table : Lookup_n-D  BreakpointsForDimension1=d_current_d_Flux  BreakpointsForDimension2=q_current_d_Flux  BreakpointsForDimension3=[5, 7]  Table=Flux_d  InternalRulePriority=Speed  RndMeth=Simplest
      settings: InputPortMap=u0,u1
  Flux_d Lookup Table1 : Lookup_n-D  BreakpointsForDimension1=d_current_d_Flux  BreakpointsForDimension2=q_current_d_Flux  BreakpointsForDimension3=[5, 7]  Table=Flux_d  InternalRulePriority=Speed  RndMeth=Simplest
      settings: InputPortMap=u0,u1
  Flux_q Lookup Table1 : Lookup_n-D  BreakpointsForDimension1=d_current_q_Flux  BreakpointsForDimension2=q_current_q_Flux  BreakpointsForDimension3=[5, 7]  Table=Flux_q  InternalRulePriority=Speed  RndMeth=Simplest
      settings: InputPortMap=u0,u1
  Flux_q Lookup Table2 : Lookup_n-D  BreakpointsForDimension1=d_current_q_Flux  BreakpointsForDimension2=q_current_q_Flux  BreakpointsForDimension3=[5, 7]  Table=Flux_q  InternalRulePriority=Speed  RndMeth=Simplest
      settings: InputPortMap=u0,u1
  Ldq Lookup Table : Lookup_n-D  BreakpointsForDimension1=d_current_q_Flux  BreakpointsForDimension2=q_current_q_Flux  BreakpointsForDimension3=[5, 7]  Table=Ldq  ExtrapMethod=Clip  UseLastTableValue=on  InternalRulePriority=Speed  OutDataTypeStr=Inherit: Inherit from 'Table data'  RndMeth=Simplest
      settings: InputPortMap=u0,u1
  Lqd Lookup Table1 : Lookup_n-D  BreakpointsForDimension1=d_current_q_Flux  BreakpointsForDimension2=q_current_q_Flux  BreakpointsForDimension3=[5, 7]  Table=Ldq  ExtrapMethod=Clip  UseLastTableValue=on  InternalRulePriority=Speed  OutDataTypeStr=Inherit: Inherit from 'Table data'  RndMeth=Simplest
      settings: InputPortMap=u0,u1
  Scope : Scope  NumInputPorts=4
  psi_d_set : Outport
  psi_q_set : Outport  Port=2
  psi_d_LUT : Outport  Port=3
  psi_q_LUT : Outport  Port=4
  Ldq_LUT : Outport  Port=5
  Lqd_LUT : Outport  Port=6
  wires:
  I_q/1 -> Flux_d Lookup Table/2, Flux_d Lookup Table1/2, Flux_q Lookup Table1/2, Ldq Lookup Table/2, Lqd Lookup Table1/2, Scope/4
  I_d/1 -> Flux_d Lookup Table/1, Flux_q Lookup Table1/1, Ldq Lookup Table/1, Lqd Lookup Table1/1, Flux_q Lookup Table2/1, Scope/3
  Lqd Lookup Table1/1 -> Lqd_LUT/1  "Ldq_Karte"
  Ldq Lookup Table/1 -> Ldq_LUT/1  "Ldq_Karte"
  Flux_q Lookup Table1/1 -> psi_q_LUT/1  "psi_q_controller"
  Flux_d Lookup Table/1 -> psi_d_LUT/1  "psi_d_controller"
  Flux_q Lookup Table2/1 -> psi_q_set/1  "psi_q_set"
  Flux_d Lookup Table1/1 -> psi_d_set/1  "psi_d_set"
  I_q_set/1 -> Flux_q Lookup Table2/2, Scope/2
  I_d_set/1 -> Flux_d Lookup Table1/1, Scope/1

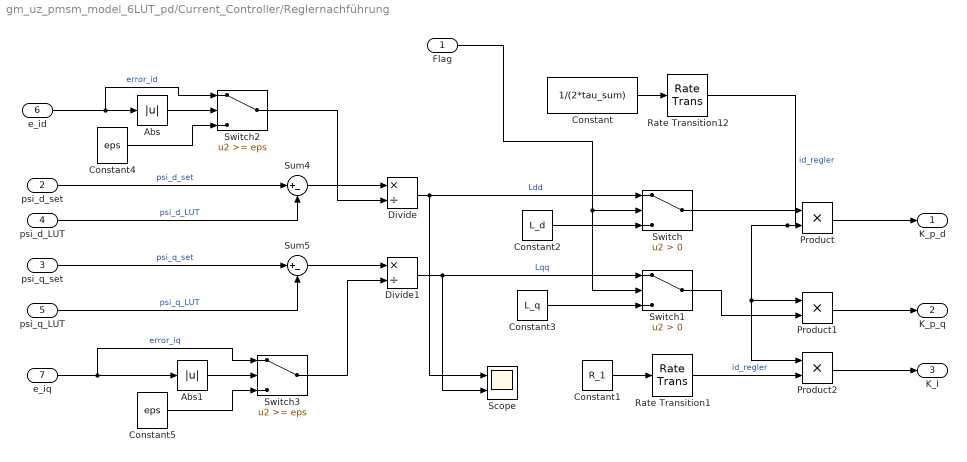
== system gm_uz_pmsm_model_6LUT_pd/Current_Controller/Reglernachführung ==
  Flag : Inport
  psi_d_set : Inport  Port=2
  psi_q_set : Inport  Port=3
  psi_d_LUT : Inport  Port=4
  psi_q_LUT : Inport  Port=5
  e_id : Inport  Port=6
  e_iq : Inport  Port=7
  Abs : Abs  SaturateOnIntegerOverflow=off
  Abs1 : Abs  SaturateOnIntegerOverflow=off
  Constant : Constant  Value=1/(2*tau_sum)
  Constant1 : Constant  Value=R_1
  Constant2 : Constant  Value=L_d
  Constant3 : Constant  Value=L_q
  Constant4 : Constant  Value=eps  SampleTime=ts_regler
  Constant5 : Constant  Value=eps  SampleTime=ts_regler
  Divide : Product  Inputs=*/
  Divide1 : Product  Inputs=*/
  Product : Product
  Product1 : Product
  Product2 : Product
  Rate Transition1 : RateTransition  OutPortSampleTime=ts_regler
  Rate Transition12 : RateTransition  OutPortSampleTime=ts_regler
  Scope : Scope  NumInputPorts=2
  Sum4 : Sum  Inputs=|+-
  Sum5 : Sum  Inputs=|+-
  Switch : Switch  Criteria=u2 > Threshold  SaturateOnIntegerOverflow=off  InputSameDT=off
  Switch1 : Switch  Criteria=u2 > Threshold  SaturateOnIntegerOverflow=off  InputSameDT=off
  Switch2 : Switch  Threshold=eps  SaturateOnIntegerOverflow=off  InputSameDT=off
  Switch3 : Switch  Threshold=eps  SaturateOnIntegerOverflow=off  InputSameDT=off
  K_p_d : Outport
  K_p_q : Outport  Port=2
  K_I : Outport  Port=3
  wires:
  Constant5/1 -> Switch3/3
  Abs1/1 -> Switch3/2
  Switch3/1 -> Divide1/2
  e_iq/1 -> Abs1/1, Switch3/1  "error_iq"
  Switch2/1 -> Divide/2
  Abs/1 -> Switch2/2
  Constant4/1 -> Switch2/3
  e_id/1 -> Abs/1, Switch2/1  "error_id"
  Divide1/1 -> Switch1/1, Scope/2  "Lqq"
  Divide/1 -> Switch/1, Scope/1  "Ldd"
  psi_q_set/1 -> Sum5/1  "psi_q_set"
  psi_d_set/1 -> Sum4/1  "psi_d_set"
  psi_d_LUT/1 -> Sum4/2  "psi_d_LUT"
  Sum5/1 -> Divide1/1
  psi_q_LUT/1 -> Sum5/2  "psi_q_LUT"
  Sum4/1 -> Divide/1
  Switch1/1 -> Product1/2
  Constant3/1 -> Switch1/3
  Switch/1 -> Product/1
  Constant2/1 -> Switch/3
  Flag/1 -> Switch1/2, Switch/2
  Rate Transition1/1 -> Product2/2  "id_regler"
  Rate Transition12/1 -> Product/2, Product1/1, Product2/1  "id_regler"
  Constant1/1 -> Rate Transition1/1
  Product2/1 -> K_I/1
  Product1/1 -> K_p_q/1
  Product/1 -> K_p_d/1
  Constant/1 -> Rate Transition12/1

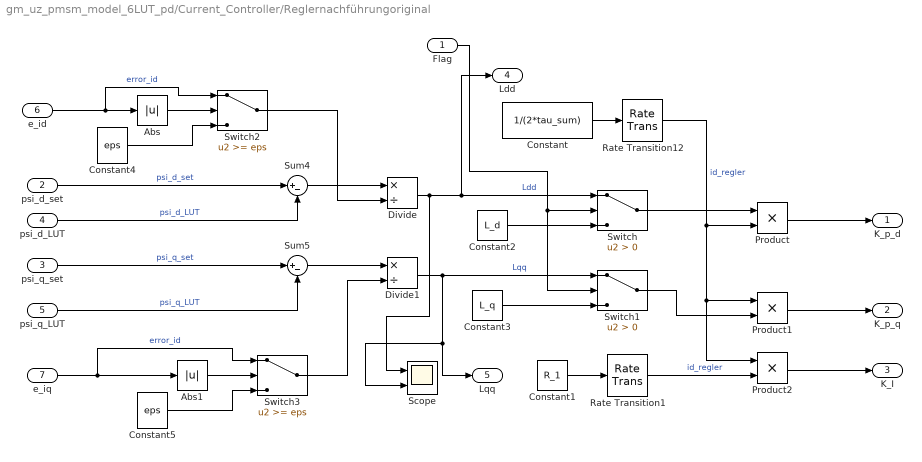
== system gm_uz_pmsm_model_6LUT_pd/Current_Controller/Reglernachführungoriginal ==
  Flag : Inport
  psi_d_set : Inport  Port=2
  psi_q_set : Inport  Port=3
  psi_d_LUT : Inport  Port=4
  psi_q_LUT : Inport  Port=5
  e_id : Inport  Port=6
  e_iq : Inport  Port=7
  Abs : Abs  SaturateOnIntegerOverflow=off
  Abs1 : Abs  SaturateOnIntegerOverflow=off
  Constant : Constant  Value=1/(2*tau_sum)
  Constant1 : Constant  Value=R_1
  Constant2 : Constant  Value=L_d
  Constant3 : Constant  Value=L_q
  Constant4 : Constant  Value=eps  SampleTime=ts_regler
  Constant5 : Constant  Value=eps  SampleTime=ts_regler
  Divide : Product  Inputs=*/
  Divide1 : Product  Inputs=*/
  Product : Product
  Product1 : Product
  Product2 : Product
  Rate Transition1 : RateTransition  OutPortSampleTime=ts_regler
  Rate Transition12 : RateTransition  OutPortSampleTime=ts_regler
  Scope : Scope  NumInputPorts=2
  Sum4 : Sum  Inputs=|+-
  Sum5 : Sum  Inputs=|+-
  Switch : Switch  Criteria=u2 > Threshold  SaturateOnIntegerOverflow=off  InputSameDT=off
  Switch1 : Switch  Criteria=u2 > Threshold  SaturateOnIntegerOverflow=off  InputSameDT=off
  Switch2 : Switch  Threshold=eps  SaturateOnIntegerOverflow=off  InputSameDT=off
  Switch3 : Switch  Threshold=eps  SaturateOnIntegerOverflow=off  InputSameDT=off
  K_p_d : Outport
  K_p_q : Outport  Port=2
  K_I : Outport  Port=3
  Ldd : Outport  Port=4
  Lqq : Outport  Port=5
  wires:
  Constant5/1 -> Switch3/3
  Abs1/1 -> Switch3/2
  Switch3/1 -> Divide1/2
  e_iq/1 -> Abs1/1, Switch3/1  "error_id"
  Switch2/1 -> Divide/2
  Abs/1 -> Switch2/2
  Constant4/1 -> Switch2/3
  e_id/1 -> Abs/1, Switch2/1  "error_id"
  Divide1/1 -> Switch1/1, Lqq/1, Scope/2  "Lqq"
  Divide/1 -> Switch/1, Ldd/1, Scope/1  "Ldd"
  psi_q_set/1 -> Sum5/1  "psi_q_set"
  psi_d_set/1 -> Sum4/1  "psi_d_set"
  psi_d_LUT/1 -> Sum4/2  "psi_d_LUT"
  Sum5/1 -> Divide1/1
  psi_q_LUT/1 -> Sum5/2  "psi_q_LUT"
  Sum4/1 -> Divide/1
  Switch1/1 -> Product1/2
  Constant3/1 -> Switch1/3
  Switch/1 -> Product/1
  Constant2/1 -> Switch/3
  Flag/1 -> Switch1/2, Switch/2
  Rate Transition1/1 -> Product2/2  "id_regler"
  Rate Transition12/1 -> Product/2, Product1/1, Product2/1  "id_regler"
  Constant1/1 -> Rate Transition1/1
  Product2/1 -> K_I/1
  Product1/1 -> K_p_q/1
  Product/1 -> K_p_d/1
  Constant/1 -> Rate Transition12/1

== system gm_uz_pmsm_model_6LUT_pd/uz_pmsm_model_6LUT/Abs ==
  In1 : Inport
  Abs : Abs  SampleTime=1e-08  OutDataTypeStr=single  SaturateOnIntegerOverflow=off
  Out1 : Outport
  wires:
  In1/1 -> Abs/1
  Abs/1 -> Out1/1

== system gm_uz_pmsm_model_6LUT_pd/uz_pmsm_model_6LUT/Data Type Conversion171 ==
  In1 : Inport
  Data Type Conversion171 : DataTypeConversion  OutDataTypeStr=single  RndMeth=Nearest  SampleTime=1e-08  SaturateOnIntegerOverflow=off
  Data Type Conversion171_pd1 : Delay  DelayLength=3
  Out1 : Outport
  wires:
  In1/1 -> Data Type Conversion171/1
  Data Type Conversion171/1 -> Data Type Conversion171_pd1/1
  Data Type Conversion171_pd1/1 -> Out1/1

== system gm_uz_pmsm_model_6LUT_pd/uz_pmsm_model_6LUT/Data Type Conversion172 ==
  In1 : Inport
  Data Type Conversion172 : DataTypeConversion  OutDataTypeStr=single  RndMeth=Nearest  SampleTime=1e-08  SaturateOnIntegerOverflow=off
  Data Type Conversion172_pd1 : Delay  DelayLength=3
  Out1 : Outport
  wires:
  In1/1 -> Data Type Conversion172/1
  Data Type Conversion172/1 -> Data Type Conversion172_pd1/1
  Data Type Conversion172_pd1/1 -> Out1/1

== system gm_uz_pmsm_model_6LUT_pd/uz_pmsm_model_6LUT/Data Type Conversion173 ==
  In1 : Inport
  Data Type Conversion173 : DataTypeConversion  OutDataTypeStr=single  RndMeth=Nearest  SampleTime=1e-08  SaturateOnIntegerOverflow=off
  Data Type Conversion173_pd1 : Delay  DelayLength=3
  Out1 : Outport
  wires:
  In1/1 -> Data Type Conversion173/1
  Data Type Conversion173/1 -> Data Type Conversion173_pd1/1
  Data Type Conversion173_pd1/1 -> Out1/1

== system gm_uz_pmsm_model_6LUT_pd/uz_pmsm_model_6LUT/Divide ==
  In1 : Inport
  In2 : Inport  Port=2
  Divide : Product  Inputs=**  OutDataTypeStr=single  SampleTime=1e-08
  Divide_pd1 : Delay  DelayLength=6
  Out1 : Outport
  wires:
  In1/1 -> Divide/1
  In2/1 -> Divide/2
  Divide/1 -> Divide_pd1/1
  Divide_pd1/1 -> Out1/1

== system gm_uz_pmsm_model_6LUT_pd/uz_pmsm_model_6LUT/Divide1 ==
  In1 : Inport
  In2 : Inport  Port=2
  Divide1 : Product  Inputs=*/  OutDataTypeStr=single  SampleTime=1e-08
  Divide1_pd1 : Delay  DelayLength=17
  Out1 : Outport
  wires:
  In1/1 -> Divide1/1
  In2/1 -> Divide1/2
  Divide1/1 -> Divide1_pd1/1
  Divide1_pd1/1 -> Out1/1

== system gm_uz_pmsm_model_6LUT_pd/uz_pmsm_model_6LUT/Divide_recip ==
  In1 : Inport
  Divide_recip : Math  Operator=reciprocal  SampleTime=1e-08
  Divide_recip_pd1 : Delay  DelayLength=16
  Out1 : Outport
  wires:
  In1/1 -> Divide_recip/1
  Divide_recip/1 -> Divide_recip_pd1/1
  Divide_recip_pd1/1 -> Out1/1

== system gm_uz_pmsm_model_6LUT_pd/uz_pmsm_model_6LUT/Factor ==
  In1 : Inport
  In2 : Inport  Port=2
  Factor : Product  Inputs=**  OutDataTypeStr=single  SampleTime=1e-08
  Factor_pd1 : Delay  DelayLength=6
  Out1 : Outport
  wires:
  In1/1 -> Factor/1
  In2/1 -> Factor/2
  Factor/1 -> Factor_pd1/1
  Factor_pd1/1 -> Out1/1

== system gm_uz_pmsm_model_6LUT_pd/uz_pmsm_model_6LUT/Gain ==
  In1 : Inport
  In2 : Inport  Port=2
  Gain : Product  Inputs=**  OutDataTypeStr=single  SampleTime=1e-08
  Gain_pd1 : Delay  DelayLength=6
  Out1 : Outport
  wires:
  In1/1 -> Gain/1
  In2/1 -> Gain/2
  Gain/1 -> Gain_pd1/1
  Gain_pd1/1 -> Out1/1

== system gm_uz_pmsm_model_6LUT_pd/uz_pmsm_model_6LUT/Gain7 ==
  In1 : Inport
  In2 : Inport  Port=2
  Gain7 : Product  Inputs=**  OutDataTypeStr=single  SampleTime=1e-08
  Gain7_pd1 : Delay  DelayLength=6
  Out1 : Outport
  wires:
  In1/1 -> Gain7/1
  In2/1 -> Gain7/2
  Gain7/1 -> Gain7_pd1/1
  Gain7_pd1/1 -> Out1/1

== system gm_uz_pmsm_model_6LUT_pd/uz_pmsm_model_6LUT/Gain71 ==
  In1 : Inport
  In2 : Inport  Port=2
  Gain71 : Product  Inputs=**  OutDataTypeStr=single  SampleTime=1e-08
  Gain71_pd1 : Delay  DelayLength=6
  Out1 : Outport
  wires:
  In1/1 -> Gain71/1
  In2/1 -> Gain71/2
  Gain71/1 -> Gain71_pd1/1
  Gain71_pd1/1 -> Out1/1

== system gm_uz_pmsm_model_6LUT_pd/uz_pmsm_model_6LUT/Gain_unaryminus ==
  In1 : Inport
  Gain_unaryminus : UnaryMinus  SampleTime=1e-08
  Out1 : Outport
  wires:
  In1/1 -> Gain_unaryminus/1
  Gain_unaryminus/1 -> Out1/1

== system gm_uz_pmsm_model_6LUT_pd/uz_pmsm_model_6LUT/Gain_unaryminus1 ==
  In1 : Inport
  Gain_unaryminus1 : UnaryMinus  SampleTime=1e-08
  Out1 : Outport
  wires:
  In1/1 -> Gain_unaryminus1/1
  Gain_unaryminus1/1 -> Out1/1
